simulink model "closed_loop1_simulink"  (R2021b)
settings: Solver=VariableStepAuto  StartTime=0.0  StopTime=15  RelTol=1e-3
values from neighbouring files (symbols this model uses):
  C = I4(1:2,:)    [open_loop.m]
  D = zeros(2,1)    [open_loop.m]
undefined symbols (not defined in the file or in its folder): A, B, K
settings Model: Creator=pieter  LastModifiedBy=pieter

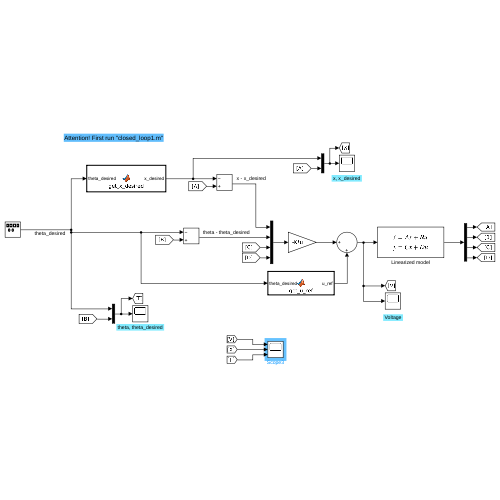
[thumbnail: Simulink's stored preview of the top-level diagram]
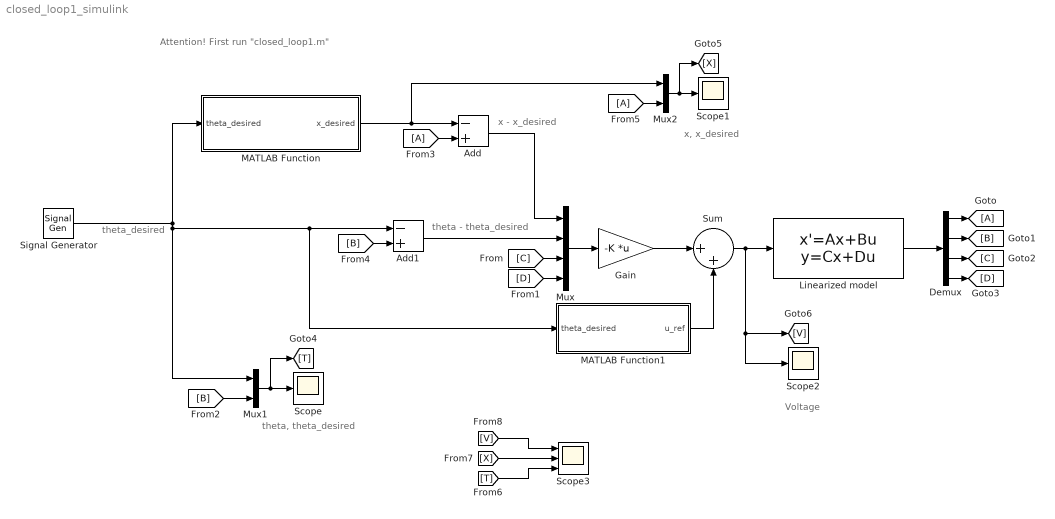
== system closed_loop1_simulink ==
  note: x, x_desired
  note: theta_desired
  note: x - x_desired
  note: theta - theta_desired
  note: Attention! First run "closed_loop1.m"
  note: theta, theta_desired
  note: Voltage
  Add : Sum  Inputs=-+
  Add1 : Sum  Inputs=-+
  Demux : Demux
  Gain : Gain  Gain=-K  Multiplication=Matrix(K*u)
  Linearized model : StateSpace  A=A  B=B  C=C  D=D  InitialCondition=0
  MATLAB Function : MATLAB Function  TreatAsAtomicUnit=on
  MATLAB Function1 : MATLAB Function  TreatAsAtomicUnit=on
  Mux : Mux
  Mux1 : Mux  Inputs=2
  Mux2 : Mux  Inputs=2
  Scope : Scope
  Scope1 : Scope
  Scope2 : Scope
  Scope3 : Scope  NumInputPorts=3
  Signal Generator : SignalGenerator  WaveForm=square  Amplitude=pi/180*5  Frequency=.10
  Sum : Sum  Inputs=|++
  wires:
  Mux/1 -> Gain/1
  [D] -> Mux/4
  [C] -> Mux/3
  Add/1 -> Mux/1
  Add1/1 -> Mux/2
  MATLAB Function/1(x_desired) -> Mux2/1, Add/1
  Signal Generator/1 -> Mux1/1, MATLAB Function1/1(theta_desired), Add1/1, MATLAB Function/1(theta_desired)
  Mux1/1 -> [T], Scope/1
  [A] -> Add/2
  [B] -> Add1/2
  Demux/1 -> [A]
  Demux/2 -> [B]
  Demux/3 -> [C]
  Demux/4 -> [D]
  [B] -> Mux1/2
  Linearized model/1 -> Demux/1
  [A] -> Mux2/2
  Mux2/1 -> [X], Scope1/1
  Gain/1 -> Sum/1
  Sum/1 -> Linearized model/1, Scope2/1, [V]
  MATLAB Function1/1(u_ref) -> Sum/2
  [V] -> Scope3/1
  [X] -> Scope3/2
  [T] -> Scope3/3

== matlab function closed_loop1_simulink/MATLAB Function ==
  data: theta_desired input; x_desired output
function x_desired = get_x_desired(theta_desired)
    Mc = 0.52;
    Msw = 3.6;
    Dt = 0.1250;
    Dc = 0.058;
    % From equation (13)
    x_desired = (Mc*Dt+Msw*Dc)*tan(theta_desired)/Mc;
end

== matlab function closed_loop1_simulink/MATLAB Function1 ==
  data: theta_desired input; u_ref output
function u_ref = get_u_ref(theta_desired)
Mc = 0.52;
g = 9.81;
F = Mc*g*sin(theta_desired);
Kt = 0.00767;
Kg = 3.71;
eta_m = 1;
eta_g = 1;
Rm = 2.6;
r = 0.00635;
u_ref = Rm*r/(eta_m*eta_g*Kt*Kg)*F;
